simulink model "SINGLE_PAHSE_INVERTER_R_LOAD"  (R2021a)
settings: Solver=VariableStepAuto  StartTime=0.0  StopTime=10  RelTol=1e-3
libraries: spsDiodeLib x4, spsMosfetLib x4, spsSeriesRLCBranchLib x3, spsVoltageMeasurementLib x2, spsDCVoltageSourceLib x1, simulink x1, spsCurrentMeasurementLib x1, spspowerguiLib x1
settings Model: Creator=vishw  LastModifiedBy=vishw

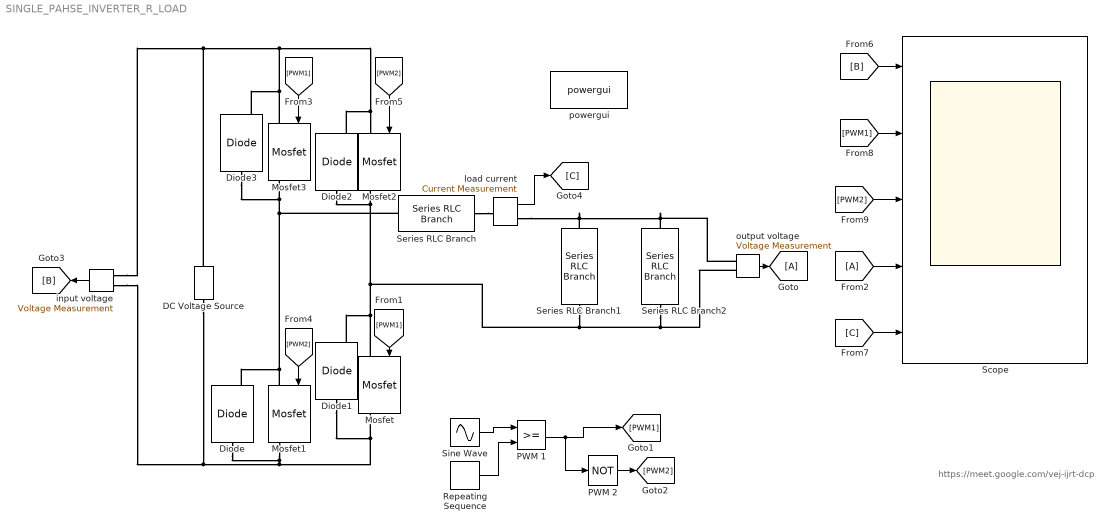
== system SINGLE_PAHSE_INVERTER_R_LOAD ==
  note: https://meet.google.com/vej-ijrt-dcp
  DC Voltage Source : spsDCVoltageSourceLib/DC Voltage Source  Amplitude=30  Measurements=None
  Diode{,1..3} (4 alike) : spsDiodeLib/Diode  Ron=0.001  Lon=0  Vf=0.8  IC=0  UseSnubber=0  Rs=500  Cs=250e-9  Measurements=on
  Mosfet{,1..3} (4 alike) : spsMosfetLib/Mosfet  Ron=0.1  Lon=0  Rd=0.01  Vfd=0  IC=0  Rs=1e5  Cs=inf  Measurements=on
  PWM 1 : RelationalOperator  OutDataTypeStr=boolean  RndMeth=Simplest
  PWM 2 : Logic  Operator=NOT  AllPortsSameDT=off  OutDataTypeStr=boolean
  Repeating Sequence : simulink/Sources/Repeating Sequence  rep_seq_t=[0 0.5]  rep_seq_y=[0 0.5]
  Scope : Scope  NumInputPorts=5
  Series RLC Branch : spsSeriesRLCBranchLib/Series RLC Branch  LConnTagsString=__new0  RConnTagsString=__new0  BranchType=L  Resistance=1  Inductance=0.5e-3  SetiL0=off  InitialCurrent=0  Capacitance=1e-6  Setx0=off  InitialVoltage=0  Measurements=None
  Series RLC Branch1 : spsSeriesRLCBranchLib/Series RLC Branch  LConnTagsString=__new0  RConnTagsString=__new0  BranchType=C  Resistance=10  Inductance=1e-3  SetiL0=off  InitialCurrent=0  Capacitance=1e-6  Setx0=off  InitialVoltage=0  Measurements=None
  Series RLC Branch2 : spsSeriesRLCBranchLib/Series RLC Branch  LConnTagsString=__new0  RConnTagsString=__new0  BranchType=R  Resistance=10  Inductance=1e-3  SetiL0=off  InitialCurrent=0  Capacitance=1e-6  Setx0=off  InitialVoltage=0  Measurements=None
  Sine Wave : Sin  SampleTime=0
  input voltage : spsVoltageMeasurementLib/Voltage Measurement  PhasorSimulation=off  OutputType=Complex  PSBequivalent=0
  load current : spsCurrentMeasurementLib/Current Measurement  PhasorSimulation=off  OutputType=Complex  PSBequivalent=0
  output voltage : spsVoltageMeasurementLib/Voltage Measurement  PhasorSimulation=off  OutputType=Complex  PSBequivalent=0
  powergui : spspowerguiLib/powergui  Priority=1  SimulationMode=Continuous  SampleTime=50e-6  frequency=60  Iterations=50  frequencyindice=0  Pbase=100e6  ErrMax=1e-4  UnitsV=kV  UnitsW=MW  buscounter=0  FunctionMessages=off  echomessages=off  EnableUseOfTLC=off  CurrentSourceSwitches=off  DisableSnubberDevices=off  DisableRonSwitches=off  DisableVfSwitches=off  DisplayEquations=off  AutomaticDiscreteSolvers=off  SolverType=Tustin/Backward Euler (TBE)  Interpol=off  ExternalGateDelay=off  methode=off  Ts=100  x0status=blocks  SPID=on  SwTol=0  HookPort=off  NonlinearTolerance=1e-4  nMaxIteration=100  ContinueOnMaxIteration=off  RestoreLinks=warning  ResistiveCurrentMeasurement=off  Frange=[0:2:500]  Ylog=off  Xlog=on  ShowGrid=off  save=off  variable=ZData  structure=0  ZoomFFT=off  StartTime=0.0  cycles=1  DisplayStyle=1  fundamental=60  FreqAxis=off  MaxFrequency=1000  frequencyindicesteady=1  RmsSteady=1  display=off
  wires:
  [PWM1] -> Mosfet3/1
  [PWM2] -> Mosfet2/1
  [PWM2] -> Mosfet1/1
  [PWM1] -> Mosfet/1
  output voltage/1 -> [A]
  input voltage/1 -> [B]
  load current/1 -> [C]
  PWM 2/1 -> [PWM2]
  [B] -> Scope/1
  [PWM1] -> Scope/2
  [PWM2] -> Scope/3
  [A] -> Scope/4
  [C] -> Scope/5
  Sine Wave/1 -> PWM 1/1
  Repeating Sequence/1 -> PWM 1/2
  PWM 1/1 -> PWM 2/1, [PWM1]
  connections:
  Mosfet3/LConn1 -- Diode3/RConn1 -- DC Voltage Source/RConn1 -- input voltage/LConn1 -- Diode2/RConn1 -- Mosfet2/LConn1
  Mosfet1/RConn1 -- Diode/LConn1 -- DC Voltage Source/LConn1 -- input voltage/LConn2 -- Diode1/LConn1 -- Mosfet/RConn1
  Mosfet1/LConn1 -- Diode/RConn1 -- Series RLC Branch/LConn1 -- Diode3/LConn1 -- Mosfet3/RConn1
  Series RLC Branch/RConn1 -- load current/LConn1
  load current/RConn1 -- Series RLC Branch1/LConn1 -- output voltage/LConn1 -- Series RLC Branch2/LConn1
  Mosfet/LConn1 -- Diode1/RConn1 -- Series RLC Branch1/RConn1 -- output voltage/LConn2 -- Series RLC Branch2/RConn1 -- Diode2/LConn1 -- Mosfet2/RConn1
